simulink model "t_t_200_tge4"  (Simulink 6.2)
settings: Solver=ode45  StartTime=0.0  StopTime=10  RelTol=1e-3
undefined symbols (not defined in the file): BEE2_usr
libraries: xbsIndex_r3 x606, xps_library x57, casper_library x22
(part 2 of 4)

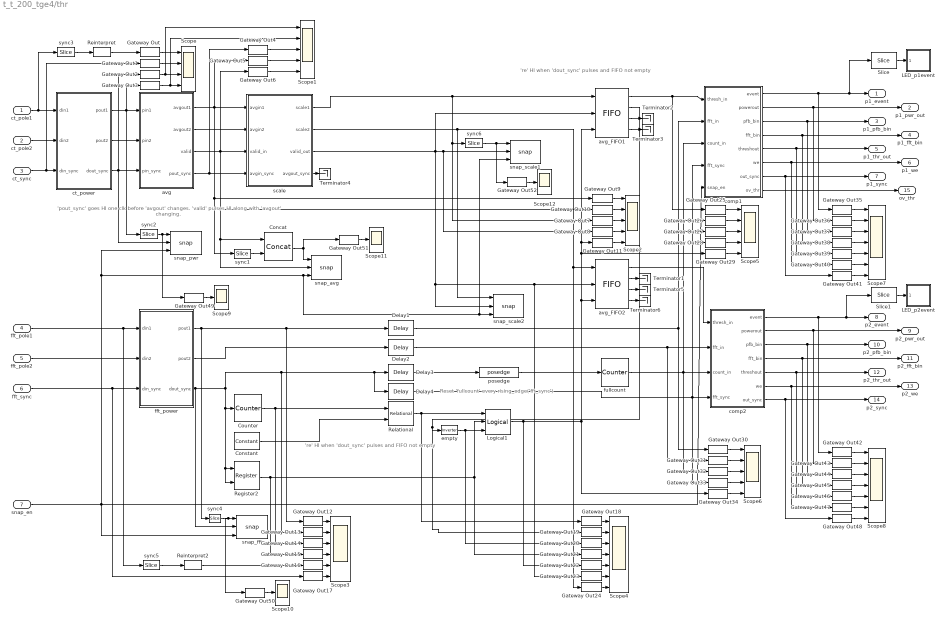
== system t_t_200_tge4/thr ==
  note: 'pout_sync' goes HI one clk
      | before 'avgout' changes.
      | 'valid' pulses HI along with
      | 'avgout' changing.
  note: 're' HI when 'dout_sync'
      | pulses and FIFO not empty
  note: 're' HI when 'dout_sync'
      | pulses and FIFO not empty
  note: Reset 'fullcount' every rising_edge('fft_sync')
  ct_pole1 : Inport  Port=1  LatchInput=off
  ct_pole2 : Inport  Port=2  LatchInput=off
  ct_sync : Inport  Port=3  LatchInput=off
  fft_pole1 : Inport  Port=4  LatchInput=off
  fft_pole2 : Inport  Port=5  LatchInput=off
  fft_sync : Inport  Port=6  LatchInput=off
  "snap_en " : Inport  Port=7  LatchInput=off
  Concat : xbsIndex_r3/Concat  num_inputs=2  explicit_period=off  period=1  dbl_ovrd=off
  Constant : xbsIndex_r3/Constant  const=0  equ=P=C  arith_type=Unsigned  n_bits=FFTSize  bin_pt=0  opselect=C  inp2=PCIN>>17  opr=+  inp1=P  carry=CIN  iostate=0  explicit_period=off  period=1  dbl_ovrd=off
  Counter : xbsIndex_r3/Counter  cnt_type=Free Running  n_bits=FFTSize  bin_pt=0  arith_type=Unsigned  start_count=0  cnt_to=Inf  cnt_by_val=1  operation=Up  explicit_period=off  period=1  load_pin=off  rst=on  en=off  dbl_ovrd=off  show_param=off  use_rpm=on  gen_core=off
      settings: xl_area=[0, 0, 0, 0, 0, 0, 0]
  Delay1 : xbsIndex_r3/Delay  latency=2  reg_retiming=off  explicit_period=off  period=1  en=off  accept_only_valid=off  init_zero=on  dbl_ovrd=off  show_param=off
      settings: xl_area=[0, 0, 0, 0, 0, 0, 0]
  Delay2 : xbsIndex_r3/Delay  latency=2  reg_retiming=off  explicit_period=off  period=1  en=off  accept_only_valid=off  init_zero=on  dbl_ovrd=off  show_param=off
      settings: xl_area=[0, 0, 0, 0, 0, 0, 0]
  Delay3 : xbsIndex_r3/Delay  latency=1  reg_retiming=off  explicit_period=off  period=1  en=off  accept_only_valid=off  init_zero=on  dbl_ovrd=off  show_param=off
      settings: xl_area=[0, 0, 0, 0, 0, 0, 0]
  Delay4 : xbsIndex_r3/Delay  latency=2  reg_retiming=off  explicit_period=off  period=1  en=off  accept_only_valid=off  init_zero=on  dbl_ovrd=off  show_param=off
      settings: xl_area=[0, 0, 0, 0, 0, 0, 0]
  Gateway Out{,1..52} (53 alike) : xbsIndex_r3/Gateway Out  output_type=Double  nbits=8  bin_pt=6  arith_type=Boolean  quantization=Truncate  overflow=Wrap  hdl_port=off  timing_constraint=None  locs_specified=off  LOCs={}  needs_fixed_name=off  show_param=off
      settings: xl_area=[0, 0, 0, 0, 0, 0, 0]
  LED_p1event : Subsystem  mask{pulse_length=200000}
      mask prompts: pulse_length "Pulse Length (samples)"
  LED_p2event : Subsystem  mask{pulse_length=200000}
      mask prompts: pulse_length "Pulse Length (samples)"
  Logical1 : xbsIndex_r3/Logical  logical_function=AND  inputs=3  precision=Full  arith_type=Unsigned  n_bits=8  bin_pt=2  align_bp=on  latency=0  explicit_period=off  period=1  en=off  dbl_ovrd=off  show_param=off
      settings: xl_area=[0, 0, 0, 0, 0, 0, 0]
  Register2 : xbsIndex_r3/Register  init=0  reg_only_valid=off  explicit_period=off  period=1  rst=off  en=on  out_en=off  dbl_ovrd=off  show_param=off
      settings: xl_area=[0, 0, 0, 0, 0, 0, 0]
  Reinterpret : xbsIndex_r3/Reinterpret  force_arith_type=on  arith_type="Signed  (2's comp)"  force_bin_pt=on  bin_pt=DataWidth-1  force_valid=on
  Reinterpret2 : xbsIndex_r3/Reinterpret  force_arith_type=on  arith_type="Signed  (2's comp)"  force_bin_pt=on  bin_pt=DataWidth-1  force_valid=on
  Relational : xbsIndex_r3/Relational  mode=a=b  latency=1  explicit_period=off  period=1  en=off  dbl_ovrd=off  show_param=off
      settings: xl_area=[0, 0, 0, 0, 0, 0, 0]
  Scope : Scope  NumInputPorts=4
      settings: YMin=-5~-5~-5~-5  YMax=5~5~5~5  SaveName=ScopeData9
  Scope{1..2,5..6} (4 alike) : Scope  NumInputPorts=5
      Scope1 settings: YMin=-5~-5~-5~-5~-5  YMax=5~5~5~5~5  SaveName=ScopeData10
      Scope2 settings: TimeRange=4300  YMin=-5~-5~-5~-5~-5  YMax=5~5~5~5~5  SaveName=ScopeData12
      Scope5 settings: YMin=-5~-5~-5~-5~-5  YMax=5~5~5~5~5  SaveName=ScopeData15
      Scope6 settings: YMin=-5~-5~-5~-5~-5  YMax=5~5~5~5~5  SaveName=ScopeData16
  Scope{9..12} (4 alike) : Scope
      Scope10 settings: YMin=8.97459e+008  YMax=9.91929e+008  SaveName=ScopeData23
      Scope11 settings: YMin=8.97459e+008  YMax=9.91929e+008  SaveName=ScopeData24
      Scope12 settings: YMin=8.97459e+008  YMax=9.91929e+008  SaveName=ScopeData25
      Scope9 settings: YMin=9.44694e+008  YMax=9.44694e+008  SaveName=ScopeData22
  Scope3 : Scope  NumInputPorts=6
      settings: YMin=-5~-5~-5~-5~-5~-5  YMax=5~5~5~5~5~5  SaveName=ScopeData13
  Scope4 : Scope  NumInputPorts=7
      settings: YMin=-5~-5~-5~-5~-5~-5~-5  YMax=5~5~5~5~5~5~5  SaveName=ScopeData14
  Scope7 : Scope  NumInputPorts=7
      settings: YMin=0~0~-1~0~0~0~0  YMax=1~1~1~1250~0.5~1~1  SaveName=ScopeData17
  Scope8 : Scope  NumInputPorts=7
      settings: YMin=-5~-5~-5~-5~-5~-5~-5  YMax=5~5~5~5~5~5~5  SaveName=ScopeData18
  Slice : xbsIndex_r3/Slice  mode=Lower Bit Location + Width  nbits=1  bit1=0  base1=MSB of Input  bit0=0  base0=LSB of Input  boolean_output=on  explicit_period=off  period=1  dbl_ovrd=off
  Slice1 : xbsIndex_r3/Slice  mode=Lower Bit Location + Width  nbits=1  bit1=0  base1=MSB of Input  bit0=0  base0=LSB of Input  boolean_output=on  explicit_period=off  period=1  dbl_ovrd=off
  Terminator{1..6} (6 alike) : Terminator
  avg : Subsystem  mask{FFTSize=FFTSize, DataWidth=DataWidth}
      mask prompts: FFTSize "FFT Size (2^?)"; DataWidth "Data Bitwidth"
  avg_FIFO1 : xbsIndex_r3/FIFO  depth=32  percent_nbits=1  store_only_valid=on  init_zero=on  explicit_period=off  period=1  rst=off  en=off  use_almost_empty=off  almost_empty_offset=6  use_almost_full=off  almost_full_offset=6  dbl_ovrd=off  show_param=off  mem_type=Block RAM  gen_core=off
      settings: xl_area=[0, 0, 0, 0, 0, 0, 0]
  avg_FIFO2 : xbsIndex_r3/FIFO  depth=32  percent_nbits=1  store_only_valid=on  init_zero=on  explicit_period=off  period=1  rst=off  en=off  use_almost_empty=off  almost_empty_offset=6  use_almost_full=off  almost_full_offset=6  dbl_ovrd=off  show_param=off  mem_type=Block RAM  gen_core=off
      settings: xl_area=[0, 0, 0, 0, 0, 0, 0]
  comp1 : Subsystem  mask{CPUWidth=CPUWidth, FFTSize=FFTSize, PFBSize=PFBSize}
      mask prompts: CPUWidth "CPU Bitwidth"; FFTSize "FFT Size (2^?)"; PFBSize "PFB Size  (2^?)"
  comp2 : Subsystem  mask{CPUWidth=CPUWidth, FFTSize=FFTSize, PFBSize=PFBSize}
      mask prompts: CPUWidth "CPU Bitwidth"; FFTSize "FFT Size (2^?)"; PFBSize "PFB Size  (2^?)"
  ct_power : Subsystem  mask{mult_lat=3, add_lat=2, DataWidth=DataWidth}
      mask prompts: mult_lat "Multiply Latency"; add_lat "Add Latency"; DataWidth "Data Width"
  empty : xbsIndex_r3/Inverter  latency=0  explicit_period=on  period=1  en=off  dbl_ovrd=off  show_param=off
      settings: xl_area=[0, 0, 0, 0, 0, 0, 0]
  fft_power : Subsystem  mask{mult_lat=3, add_lat=2, DataWidth=DataWidth}
      mask prompts: mult_lat "Multiply Latency"; add_lat "Add Latency"; DataWidth "Data Width"
  fullcount : xbsIndex_r3/Counter  cnt_type=Free Running  n_bits=FFTSize+PFBSize  bin_pt=0  arith_type=Unsigned  start_count=0  cnt_to=Inf  cnt_by_val=1  operation=Up  explicit_period=off  period=1  load_pin=off  rst=on  en=off  dbl_ovrd=off  show_param=off  use_rpm=on  gen_core=off
      settings: xl_area=[0, 0, 0, 0, 0, 0, 0]
  posedge : casper_library/Misc/posedge  Tag=Rising Edge Detector
  scale : Subsystem  mask{DataWidth=DataWidth, mult_lat=4, scale=1}
      mask prompts: DataWidth "Data Bitwidth"; mult_lat "Mulitply Latency"; scale "Test Scale"
  snap_avg : casper_library/Scopes/snap  nsamples=11
  snap_fft : casper_library/Scopes/snap  nsamples=11
  snap_pwr : casper_library/Scopes/snap  nsamples=11
  snap_scale1 : casper_library/Scopes/snap  nsamples=11
  snap_scale2 : casper_library/Scopes/snap  nsamples=11
  sync1 : xbsIndex_r3/Slice  mode=Lower Bit Location + Width  nbits=31  bit1=0  base1=MSB of Input  bit0=0  base0=LSB of Input  boolean_output=off  explicit_period=off  period=1  dbl_ovrd=off
  sync2 : xbsIndex_r3/Slice  mode=Lower Bit Location + Width  nbits=32  bit1=0  base1=MSB of Input  bit0=0  base0=LSB of Input  boolean_output=off  explicit_period=off  period=1  dbl_ovrd=off
  sync3 : xbsIndex_r3/Slice  mode=Lower Bit Location + Width  nbits=DataWidth  bit1=0  base1=MSB of Input  bit0=0  base0=LSB of Input  boolean_output=off  explicit_period=off  period=1  dbl_ovrd=off
  sync4 : xbsIndex_r3/Slice  mode=Lower Bit Location + Width  nbits=DataWidth  bit1=0  base1=MSB of Input  bit0=0  base0=LSB of Input  boolean_output=off  explicit_period=off  period=1  dbl_ovrd=off
  sync5 : xbsIndex_r3/Slice  mode=Lower Bit Location + Width  nbits=DataWidth  bit1=0  base1=MSB of Input  bit0=0  base0=LSB of Input  boolean_output=off  explicit_period=off  period=1  dbl_ovrd=off
  sync6 : xbsIndex_r3/Slice  mode=Lower Bit Location + Width  nbits=32  bit1=0  base1=MSB of Input  bit0=0  base0=LSB of Input  boolean_output=off  explicit_period=off  period=1  dbl_ovrd=off
  p1_event : Outport
  p1_pwr_out : Outport  Port=2
  p1_pfb_bin : Outport  Port=3
  p1_fft_bin : Outport  Port=4
  p1_thr_out : Outport  Port=5
  p1_we : Outport  Port=6
  p1_sync : Outport  Port=7
  p2_event : Outport  Port=8
  p2_pwr_out : Outport  Port=9
  p2_pfb_bin : Outport  Port=10
  p2_fft_bin : Outport  Port=11
  p2_thr_out : Outport  Port=12
  p2_we : Outport  Port=13
  p2_sync : Outport  Port=14
  ov_thr : Outport  Port=15
  wires:
  Slice1/1 -> LED_p2event/1(Sync_In)
  Gateway Out48/1 -> Scope8/7
  Gateway Out47/1 -> Scope8/6
  Gateway Out46/1 -> Scope8/5
  Gateway Out45/1 -> Scope8/4
  Gateway Out44/1 -> Scope8/3
  Gateway Out43/1 -> Scope8/2
  Gateway Out42/1 -> Scope8/1
  Gateway Out41/1 -> Scope7/7
  Gateway Out40/1 -> Scope7/6
  Gateway Out39/1 -> Scope7/5
  Gateway Out38/1 -> Scope7/4
  Gateway Out37/1 -> Scope7/3
  Gateway Out36/1 -> Scope7/2
  Gateway Out35/1 -> Scope7/1
  Gateway Out34/1 -> Scope6/5
  Gateway Out33/1 -> Scope6/4
  Gateway Out32/1 -> Scope6/3
  Gateway Out31/1 -> Scope6/2
  Gateway Out30/1 -> Scope6/1
  Gateway Out29/1 -> Scope5/5
  Gateway Out28/1 -> Scope5/4
  Gateway Out27/1 -> Scope5/3
  Gateway Out26/1 -> Scope5/2
  Gateway Out25/1 -> Scope5/1
  Gateway Out24/1 -> Scope4/7
  Gateway Out23/1 -> Scope4/6
  Gateway Out22/1 -> Scope4/5
  Gateway Out21/1 -> Scope4/4
  Gateway Out20/1 -> Scope4/3
  Gateway Out19/1 -> Scope4/2
  Gateway Out18/1 -> Scope4/1
  Gateway Out17/1 -> Scope3/6
  Gateway Out16/1 -> Scope3/5
  Gateway Out15/1 -> Scope3/4
  Gateway Out14/1 -> Scope3/3
  Gateway Out13/1 -> Scope3/2
  Gateway Out12/1 -> Scope3/1
  Gateway Out11/1 -> Scope2/5
  Gateway Out8/1 -> Scope2/4
  Gateway Out7/1 -> Scope2/3
  Gateway Out10/1 -> Scope2/2
  Gateway Out9/1 -> Scope2/1
  Gateway Out4/1 -> Scope1/3
  Gateway Out5/1 -> Scope1/4
  Gateway Out6/1 -> Scope1/5
  Gateway Out3/1 -> Scope/4, Scope1/2
  Gateway Out2/1 -> Scope/3, Scope1/1
  Gateway Out1/1 -> Scope/2
  Gateway Out/1 -> Scope/1
  Reinterpret/1 -> Gateway Out/1
  sync3/1 -> Reinterpret/1
  ct_sync/1 -> Gateway Out1/1, ct_power/3(din_sync)
  scale/1(scale1) -> Gateway Out7/1, sync6/1, avg_FIFO1/1
  sync2/1 -> snap_pwr/1, Gateway Out49/1
  comp1/6(we) -> p1_we/1, Gateway Out40/1
  comp1/1(event) -> Gateway Out35/1, Slice/1, p1_event/1
  sync1/1 -> Concat/2
  Concat/1 -> snap_avg/1, Gateway Out51/1
  "snap_en "/1 -> snap_pwr/3, snap_avg/3, snap_scale2/3, snap_scale1/3, comp1/5("snap_en "), snap_fft/3
  scale/4(avgout_sync) -> Terminator4/1
  empty/1 -> Gateway Out20/1, Logical1/3
  Logical1/1 -> Gateway Out22/1, Gateway Out34/1, Gateway Out29/1, Gateway Out11/1, avg_FIFO1/3, avg_FIFO2/3
  avg_FIFO1/2 -> Gateway Out19/1, empty/1
  avg/4(pout_sync) -> Gateway Out4/1, scale/4(avgin_sync)
  Delay2/1 -> comp2/2(fft_in), Gateway Out31/1
  Slice/1 -> LED_p1event/1(Sync_In)
  avg/3(valid) -> Gateway Out10/1, Concat/1, snap_avg/2, Gateway Out6/1, scale/3(valid_in)
  Relational/1 -> Gateway Out18/1, Logical1/1
  Register2/1 -> Gateway Out21/1, Logical1/2, Gateway Out15/1
  fft_sync/1 -> Gateway Out17/1, fft_power/3(din_sync)
  fft_pole2/1 -> fft_power/2(din2)
  fft_pole1/1 -> fft_power/1(din1), sync5/1
  ct_pole2/1 -> ct_power/2(din2)
  ct_pole1/1 -> sync3/1, ct_power/1(din1)
  comp2/7(out_sync) -> Gateway Out48/1, p2_sync/1
  comp2/6(we) -> Gateway Out47/1, p2_we/1
  comp2/5(threshout) -> Gateway Out46/1, p2_thr_out/1
  comp2/4(fft_bin) -> Gateway Out45/1, p2_fft_bin/1
  comp2/3(pfb_bin) -> Gateway Out44/1, p2_pfb_bin/1
  comp2/2(powerout) -> Gateway Out43/1, p2_pwr_out/1
  comp2/1(event) -> Slice1/1, p2_event/1, Gateway Out42/1
  comp1/7(out_sync) -> Gateway Out41/1, p1_sync/1
  comp1/5(threshout) -> Gateway Out39/1, p1_thr_out/1
  comp1/4(fft_bin) -> Gateway Out38/1, p1_fft_bin/1
  comp1/3(pfb_bin) -> Gateway Out37/1, p1_pfb_bin/1
  comp1/2(powerout) -> Gateway Out36/1, p1_pwr_out/1
  Delay1/1 -> Gateway Out30/1, Gateway Out26/1, comp1/2(fft_in)
  fullcount/1 -> comp2/3(count_in), Gateway Out32/1, Gateway Out27/1, comp1/3(count_in)
  fft_power/2(pout2) -> Delay2/1
  avg_FIFO2/4 -> Terminator6/1
  avg_FIFO2/3 -> Terminator5/1
  avg_FIFO1/4 -> Terminator3/1
  avg_FIFO1/3 -> Terminator2/1
  avg_FIFO2/1 -> comp2/1(thresh_in)
  fft_power/1(pout1) -> Gateway Out12/1, Delay1/1, sync4/1
  avg_FIFO1/1 -> Gateway Out25/1, comp1/1(thresh_in)
  fft_power/3(dout_sync) -> Gateway Out13/1, Delay3/1, Delay4/1, Counter/1, Register2/1, Register2/2, snap_fft/2
  Constant/1 -> Relational/2
  Counter/1 -> Gateway Out14/1, Relational/1
  scale/3(valid_out) -> Gateway Out8/1, snap_scale1/2, avg_FIFO1/2, Gateway Out23/1, avg_FIFO2/2, snap_scale2/2
  scale/2(scale2) -> Gateway Out24/1, avg_FIFO2/1, snap_scale2/1
  avg/2(avgout2) -> scale/2(avgin2)
  avg/1(avgout1) -> Gateway Out9/1, sync1/1, Gateway Out5/1, scale/1(avgin1)
  ct_power/3(dout_sync) -> Gateway Out2/1, avg/3(pin_sync), snap_pwr/2
  ct_power/2(pout2) -> avg/2(pin2)
  ct_power/1(pout1) -> Gateway Out3/1, sync2/1, avg/1(pin1)
  sync5/1 -> Reinterpret2/1
  Reinterpret2/1 -> Gateway Out16/1
  Delay3/1 -> posedge/1
  posedge/1 -> fullcount/1
  Delay4/1 -> comp2/4(fft_sync), Gateway Out33/1, comp1/4(fft_sync), Gateway Out28/1
  Gateway Out49/1 -> Scope9/1
  sync4/1 -> snap_fft/1, Gateway Out50/1
  Gateway Out50/1 -> Scope10/1
  Gateway Out51/1 -> Scope11/1
  sync6/1 -> snap_scale1/1, Gateway Out52/1
  Gateway Out52/1 -> Scope12/1
  comp1/8(ov_thr) -> ov_thr/1
  avg_FIFO2/2 -> Terminator1/1

== system t_t_200_tge4/ct_in_mux/concat ==
  In1 : Inport  Orientation=down  Port=1  LatchInput=off
  Concat : xbsIndex_r3/Concat  num_inputs=4  explicit_period=on  period=1  dbl_ovrd=off
  Constant : xbsIndex_r3/Constant  const=0  equ=P=C  arith_type=Unsigned  n_bits=14  bin_pt=0  opselect=C  inp2=PCIN>>17  opr=+  inp1=P  carry=CIN  iostate=0  explicit_period=on  period=1  dbl_ovrd=off
  Slice3 : xbsIndex_r3/Slice  mode=Upper Bit Location + Width  nbits=18  bit1=0  base1=MSB of Input  bit0=0  base0=LSB of Input  boolean_output=off  explicit_period=off  period=1  dbl_ovrd=off
  Slice4 : xbsIndex_r3/Slice  mode=Lower Bit Location + Width  nbits=18  bit1=0  base1=MSB of Input  bit0=0  base0=LSB of Input  boolean_output=off  explicit_period=off  period=1  dbl_ovrd=off
  Out1 : Outport
  wires:
  Slice3/1 -> Concat/2
  Constant/1 -> Concat/1, Concat/3
  Slice4/1 -> Concat/4
  In1/1 -> Slice3/1, Slice4/1
  Concat/1 -> Out1/1

== system t_t_200_tge4/ct_in_mux/trig_delay ==
  data_in : Inport  Port=1  LatchInput=off
  trig_in : Inport  Port=2  LatchInput=off
  delay : Inport  Port=3  LatchInput=off
  Constant : xbsIndex_r3/Constant  const=1  equ=P=C  arith_type=Boolean  n_bits=32  bin_pt=0  opselect=C  inp2=PCIN>>17  opr=+  inp1=P  carry=CIN  iostate=0  explicit_period=on  period=1  dbl_ovrd=off
  Counter : xbsIndex_r3/Counter  cnt_type=Free Running  n_bits=32  bin_pt=0  arith_type=Unsigned  start_count=0  cnt_to=Inf  cnt_by_val=1  operation=Up  explicit_period=on  period=1  load_pin=off  rst=on  en=on  dbl_ovrd=off  show_param=off  use_rpm=on  gen_core=off
      settings: xl_area=[0, 0, 0, 0, 0, 0, 0]
  Delay : xbsIndex_r3/Delay  latency=2  reg_retiming=off  explicit_period=on  period=1  en=off  accept_only_valid=off  init_zero=on  dbl_ovrd=off  show_param=off
      settings: xl_area=[0, 0, 0, 0, 0, 0, 0]
  Gateway Out : xbsIndex_r3/Gateway Out  output_type=Double  nbits=8  bin_pt=6  arith_type=Boolean  quantization=Truncate  overflow=Wrap  hdl_port=on  timing_constraint=None  locs_specified=off  LOCs={}  needs_fixed_name=off  show_param=off
      settings: xl_area=[0, 0, 0, 0, 0, 0, 0]
  Gateway Out1 : xbsIndex_r3/Gateway Out  output_type=Double  nbits=8  bin_pt=6  arith_type=Boolean  quantization=Truncate  overflow=Wrap  hdl_port=on  timing_constraint=None  locs_specified=off  LOCs={}  needs_fixed_name=off  show_param=off
      settings: xl_area=[0, 0, 0, 0, 0, 0, 0]
  Register : xbsIndex_r3/Register  init=0  reg_only_valid=off  explicit_period=on  period=1  rst=on  en=on  out_en=off  dbl_ovrd=off  show_param=off
      settings: xl_area=[0, 0, 0, 0, 0, 0, 0]
  Relational : xbsIndex_r3/Relational  mode=a=b  latency=1  explicit_period=on  period=1  en=on  dbl_ovrd=off  show_param=off
      settings: xl_area=[0, 0, 0, 0, 0, 0, 0]
  Scope : Scope  NumInputPorts=2
      settings: YMin=-5~-5  YMax=5~5
  posedge : casper_library/Misc/posedge  Tag=Rising Edge Detector
  data_out : Outport
  trig_out : Outport  Port=2
  wires:
  delay/1 -> Relational/1
  trig_in/1 -> Register/3, Gateway Out1/1
  Constant/1 -> Register/1
  Relational/1 -> Register/2, Counter/1, Gateway Out/1, posedge/1
  Register/1 -> Counter/2, Relational/3
  Counter/1 -> Relational/2
  Gateway Out/1 -> Scope/1
  Gateway Out1/1 -> Scope/2
  data_in/1 -> Delay/1
  Delay/1 -> data_out/1
  posedge/1 -> trig_out/1

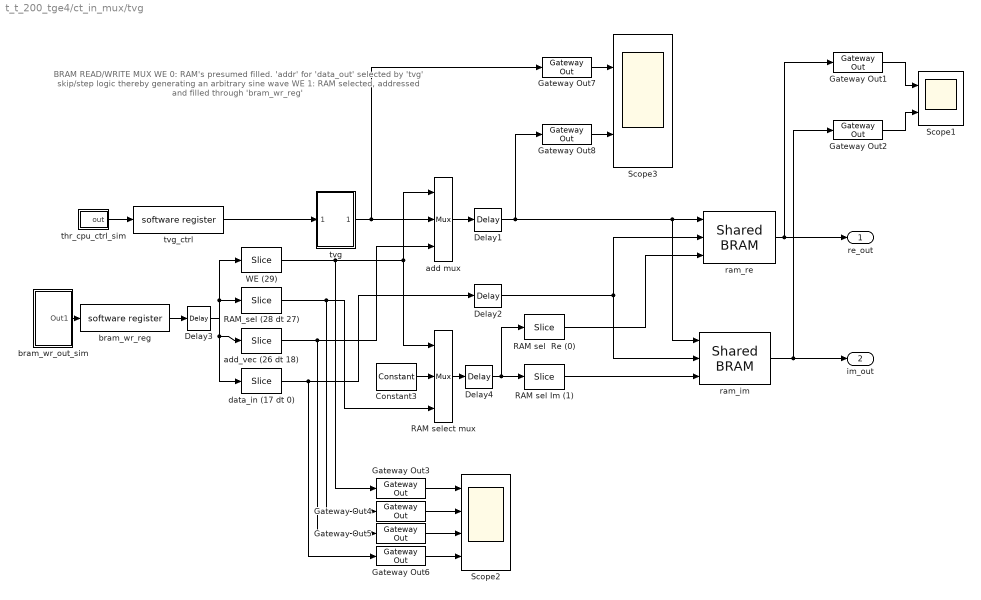
== system t_t_200_tge4/ct_in_mux/tvg ==
  note: BRAM READ/WRITE MUX
      | WE 0: RAM's presumed filled.
      | 'addr' for 'data_out' selected
      | by 'tvg' skip/step logic thereby
      | generating an arbitrary sine wave
      | WE 1: RAM selected, addressed
      | and filled through
      | 'bram_wr_reg'
  Constant3 : xbsIndex_r3/Constant  const=0  equ=P=C  arith_type=Unsigned  n_bits=4  bin_pt=0  opselect=C  inp2=PCIN>>17  opr=+  inp1=P  carry=CIN  iostate=0  explicit_period=on  period=1  dbl_ovrd=off
  Delay{1..4} (4 alike) : xbsIndex_r3/Delay  latency=1  reg_retiming=on  explicit_period=on  period=1  en=off  accept_only_valid=off  init_zero=on  dbl_ovrd=off  show_param=off
      settings: xl_area=[0, 0, 0, 0, 0, 0, 0]
  Gateway Out{1..8} (8 alike) : xbsIndex_r3/Gateway Out  output_type=Double  nbits=8  bin_pt=6  arith_type=Boolean  quantization=Truncate  overflow=Wrap  hdl_port=on  timing_constraint=None  locs_specified=off  LOCs={}  needs_fixed_name=off  show_param=off
      settings: xl_area=[0, 0, 0, 0, 0, 0, 0]
  RAM sel  Re (0) : xbsIndex_r3/Slice  mode=Lower Bit Location + Width  nbits=1  bit1=0  base1=MSB of Input  bit0=0  base0=LSB of Input  boolean_output=on  explicit_period=on  period=1  dbl_ovrd=off
  RAM sel Im (1) : xbsIndex_r3/Slice  mode=Lower Bit Location + Width  nbits=1  bit1=0  base1=MSB of Input  bit0=1  base0=LSB of Input  boolean_output=on  explicit_period=on  period=1  dbl_ovrd=off
  RAM select mux : xbsIndex_r3/Mux  inputs=2  precision=Full  arith_type="Signed  (2's comp)"  n_bits=8  bin_pt=2  quantization=Truncate  overflow=Wrap  latency=0  explicit_period=on  period=1  en=off  dbl_ovrd=off  show_param=off  mux_type=off  use_rpm=off  gen_core=off
      settings: xl_area=[0, 0, 0, 0, 0, 0, 0]
  RAM_sel (28 dt 27) : xbsIndex_r3/Slice  mode=Lower Bit Location + Width  nbits=2  bit1=10  base1=MSB of Input  bit0=27  base0=LSB of Input  boolean_output=off  explicit_period=on  period=1  dbl_ovrd=off
  Scope1 : Scope  NumInputPorts=2
      settings: YMin=-5~-5  YMax=5~5  SaveName=ScopeData2
  Scope2 : Scope  NumInputPorts=4
      settings: YMin=-5~-5~-5~-5  YMax=5~5~5~5
  Scope3 : Scope  NumInputPorts=2
      settings: YMin=-5~-5  YMax=5~5  SaveName=ScopeData3
  WE (29) : xbsIndex_r3/Slice  mode=Lower Bit Location + Width  nbits=1  bit1=10  base1=MSB of Input  bit0=29  base0=LSB of Input  boolean_output=off  explicit_period=on  period=1  dbl_ovrd=off
  add mux : xbsIndex_r3/Mux  inputs=2  precision=Full  arith_type="Signed  (2's comp)"  n_bits=8  bin_pt=2  quantization=Truncate  overflow=Wrap  latency=0  explicit_period=on  period=1  en=off  dbl_ovrd=off  show_param=off  mux_type=off  use_rpm=off  gen_core=off
      settings: xl_area=[0, 0, 0, 0, 0, 0, 0]
  add_vec (26 dt 18) : xbsIndex_r3/Slice  mode=Lower Bit Location + Width  nbits=9  bit1=0  base1=MSB of Input  bit0=18  base0=LSB of Input  boolean_output=off  explicit_period=on  period=1  dbl_ovrd=off
  bram_wr_out_sim : Subsystem  mask{we_enable=0, ram_sel=3, add_vec=512, data_in=32}
      mask prompts: we_enable "Write enable"; ram_sel "RAM selector (1 = Re; 2 = Im; 3 = both)"; add_vec "RAM address"; data_in "Data in"
  bram_wr_reg : xps_library/software register  Tag=xps:sw_reg  io_dir=From Processor  arith_type=Unsigned  bitwidth=32  bin_pt=0  sample_period=1  gw_name=t_t_200_tge4_ct_in_mux_tvg_bram_wr_reg_user_data_out
  data_in (17 dt 0) : xbsIndex_r3/Slice  mode=Lower Bit Location + Width  nbits=18  bit1=0  base1=MSB of Input  bit0=0  base0=LSB of Input  boolean_output=off  explicit_period=on  period=1  dbl_ovrd=off
  ram_im : xps_library/Shared BRAM  Tag=xps:bram  arith_type="Signed  (2's comp)"  addr_width=11  data_width=32  data_bin_pt=0  init_vals=[1:2^11]  sample_rate=1
  ram_re : xps_library/Shared BRAM  Tag=xps:bram  arith_type="Signed  (2's comp)"  addr_width=11  data_width=32  data_bin_pt=0  init_vals=[1:2^11]  sample_rate=1
  thr_cpu_ctrl_sim : Subsystem  mask{tvg_skip=1, tvg_stall=2, tvg_length=5}
      mask prompts: tvg_skip "Skip"; tvg_stall "Stall"; tvg_length "Length"
      mask help:
      | Mux Data for CT and FFT Syncs:
      |
      | 0 -> Interchip Connection
      | 1 -> User Generated External Sync
      | 2 -> Periodic Sync Generator
      | 3 -> Periodic Sync Generator (Same as 2)
      |
      | Mux Data for CT and FFT Inputs:
      |
      | 0 -> Interchip Connection
      | 1 -> Test Vector Generator (TVG)
      | 2 -> All Zeroes (0's)
      | 3 -> All Ones (1's)
  tvg : Subsystem  mask(Test Vector Generator(TVG)){tvg_skip=1, tvg_stall=1, tvg_length=512}
      mask prompts: tvg_skip "Skip"; tvg_stall "Stall"; tvg_length "Length"
  tvg_ctrl : xps_library/software register  Tag=xps:sw_reg  io_dir=From Processor  arith_type=Unsigned  bitwidth=32  bin_pt=0  sample_period=1  gw_name=t_t_200_tge4_ct_in_mux_tvg_tvg_ctrl_user_data_out
  re_out : Outport
  im_out : Outport  Port=2
  wires:
  Delay3/1 -> RAM_sel (28 dt 27)/1, WE (29)/1, add_vec (26 dt 18)/1, data_in (17 dt 0)/1
  bram_wr_reg/1 -> Delay3/1
  tvg_ctrl/1 -> tvg/1(In1)
  tvg/1(Out1) -> add mux/2, Gateway Out7/1
  Constant3/1 -> RAM select mux/2
  RAM select mux/1 -> Delay4/1
  RAM sel  Re (0)/1 -> ram_re/3
  Gateway Out1/1 -> Scope1/1
  Gateway Out2/1 -> Scope1/2
  thr_cpu_ctrl_sim/1(out) -> tvg_ctrl/1
  add_vec (26 dt 18)/1 -> Gateway Out5/1, add mux/3
  RAM_sel (28 dt 27)/1 -> Gateway Out4/1, RAM select mux/3
  add mux/1 -> Delay1/1
  data_in (17 dt 0)/1 -> Gateway Out6/1, Delay2/1
  RAM sel Im (1)/1 -> ram_im/3
  ram_re/1 -> Gateway Out1/1, re_out/1
  ram_im/1 -> Gateway Out2/1, im_out/1
  bram_wr_out_sim/1(Out1) -> bram_wr_reg/1
  Gateway Out3/1 -> Scope2/1
  Gateway Out4/1 -> Scope2/2
  Gateway Out5/1 -> Scope2/3
  Gateway Out6/1 -> Scope2/4
  WE (29)/1 -> Gateway Out3/1, add mux/1, RAM select mux/1
  Gateway Out7/1 -> Scope3/1
  Gateway Out8/1 -> Scope3/2
  Delay1/1 -> ram_im/1, ram_re/1, Gateway Out8/1
  Delay2/1 -> ram_re/2, ram_im/2
  Delay4/1 -> RAM sel  Re (0)/1, RAM sel Im (1)/1

== system t_t_200_tge4/fft_in_mux/concat ==
  In1 : Inport  Port=1  LatchInput=off
  Concat : xbsIndex_r3/Concat  num_inputs=4  explicit_period=on  period=1  dbl_ovrd=off
  Constant : xbsIndex_r3/Constant  const=0  equ=P=C  arith_type=Unsigned  n_bits=14  bin_pt=0  opselect=C  inp2=PCIN>>17  opr=+  inp1=P  carry=CIN  iostate=0  explicit_period=on  period=1  dbl_ovrd=off
  Slice3 : xbsIndex_r3/Slice  mode=Upper Bit Location + Width  nbits=18  bit1=0  base1=MSB of Input  bit0=0  base0=LSB of Input  boolean_output=off  explicit_period=off  period=1  dbl_ovrd=off
  Slice4 : xbsIndex_r3/Slice  mode=Lower Bit Location + Width  nbits=18  bit1=0  base1=MSB of Input  bit0=0  base0=LSB of Input  boolean_output=off  explicit_period=off  period=1  dbl_ovrd=off
  Out1 : Outport
  wires:
  Slice4/1 -> Concat/4
  Slice3/1 -> Concat/2
  Constant/1 -> Concat/1, Concat/3
  In1/1 -> Slice4/1, Slice3/1
  Concat/1 -> Out1/1

== system t_t_200_tge4/fft_in_mux/trig_delay ==
  data_in : Inport  Port=1  LatchInput=off
  trig_in : Inport  Port=2  LatchInput=off
  delay : Inport  Port=3  LatchInput=off
  Constant : xbsIndex_r3/Constant  const=1  equ=P=C  arith_type=Boolean  n_bits=32  bin_pt=0  opselect=C  inp2=PCIN>>17  opr=+  inp1=P  carry=CIN  iostate=0  explicit_period=on  period=1  dbl_ovrd=off
  Counter : xbsIndex_r3/Counter  cnt_type=Free Running  n_bits=32  bin_pt=0  arith_type=Unsigned  start_count=0  cnt_to=Inf  cnt_by_val=1  operation=Up  explicit_period=on  period=1  load_pin=off  rst=on  en=on  dbl_ovrd=off  show_param=off  use_rpm=on  gen_core=off
      settings: xl_area=[0, 0, 0, 0, 0, 0, 0]
  Delay : xbsIndex_r3/Delay  latency=2  reg_retiming=off  explicit_period=on  period=1  en=off  accept_only_valid=off  init_zero=on  dbl_ovrd=off  show_param=off
      settings: xl_area=[0, 0, 0, 0, 0, 0, 0]
  Gateway Out : xbsIndex_r3/Gateway Out  output_type=Double  nbits=8  bin_pt=6  arith_type=Boolean  quantization=Truncate  overflow=Wrap  hdl_port=on  timing_constraint=None  locs_specified=off  LOCs={}  needs_fixed_name=off  show_param=off
      settings: xl_area=[0, 0, 0, 0, 0, 0, 0]
  Gateway Out1 : xbsIndex_r3/Gateway Out  output_type=Double  nbits=8  bin_pt=6  arith_type=Boolean  quantization=Truncate  overflow=Wrap  hdl_port=on  timing_constraint=None  locs_specified=off  LOCs={}  needs_fixed_name=off  show_param=off
      settings: xl_area=[0, 0, 0, 0, 0, 0, 0]
  Register : xbsIndex_r3/Register  init=0  reg_only_valid=off  explicit_period=on  period=1  rst=on  en=on  out_en=off  dbl_ovrd=off  show_param=off
      settings: xl_area=[0, 0, 0, 0, 0, 0, 0]
  Relational : xbsIndex_r3/Relational  mode=a=b  latency=1  explicit_period=on  period=1  en=on  dbl_ovrd=off  show_param=off
      settings: xl_area=[0, 0, 0, 0, 0, 0, 0]
  Scope : Scope  NumInputPorts=2
      settings: YMin=-5~-5  YMax=5~5
  posedge : casper_library/Misc/posedge  Tag=Rising Edge Detector
  data_out : Outport
  trig_out : Outport  Port=2
  wires:
  delay/1 -> Relational/1
  trig_in/1 -> Register/3, Gateway Out1/1
  Constant/1 -> Register/1
  Relational/1 -> Register/2, Counter/1, Gateway Out/1, posedge/1
  Register/1 -> Counter/2, Relational/3
  Counter/1 -> Relational/2
  Gateway Out/1 -> Scope/1
  Gateway Out1/1 -> Scope/2
  data_in/1 -> Delay/1
  Delay/1 -> data_out/1
  posedge/1 -> trig_out/1

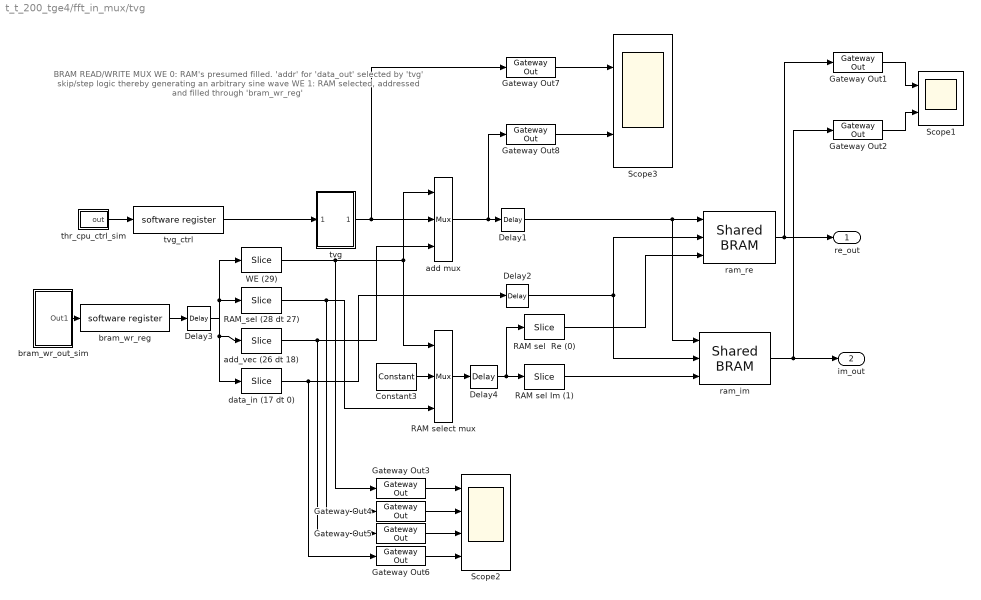
== system t_t_200_tge4/fft_in_mux/tvg ==
  note: BRAM READ/WRITE MUX
      | WE 0: RAM's presumed filled.
      | 'addr' for 'data_out' selected
      | by 'tvg' skip/step logic thereby
      | generating an arbitrary sine wave
      | WE 1: RAM selected, addressed
      | and filled through
      | 'bram_wr_reg'
  Constant3 : xbsIndex_r3/Constant  const=0  equ=P=C  arith_type=Unsigned  n_bits=4  bin_pt=0  opselect=C  inp2=PCIN>>17  opr=+  inp1=P  carry=CIN  iostate=0  explicit_period=on  period=1  dbl_ovrd=off
  Delay{1..4} (4 alike) : xbsIndex_r3/Delay  latency=1  reg_retiming=on  explicit_period=on  period=1  en=off  accept_only_valid=off  init_zero=on  dbl_ovrd=off  show_param=off
      settings: xl_area=[0, 0, 0, 0, 0, 0, 0]
  Gateway Out{1..8} (8 alike) : xbsIndex_r3/Gateway Out  output_type=Double  nbits=8  bin_pt=6  arith_type=Boolean  quantization=Truncate  overflow=Wrap  hdl_port=on  timing_constraint=None  locs_specified=off  LOCs={}  needs_fixed_name=off  show_param=off
      settings: xl_area=[0, 0, 0, 0, 0, 0, 0]
  RAM sel  Re (0) : xbsIndex_r3/Slice  mode=Lower Bit Location + Width  nbits=1  bit1=0  base1=MSB of Input  bit0=0  base0=LSB of Input  boolean_output=on  explicit_period=on  period=1  dbl_ovrd=off
  RAM sel Im (1) : xbsIndex_r3/Slice  mode=Lower Bit Location + Width  nbits=1  bit1=0  base1=MSB of Input  bit0=1  base0=LSB of Input  boolean_output=on  explicit_period=on  period=1  dbl_ovrd=off
  RAM select mux : xbsIndex_r3/Mux  inputs=2  precision=Full  arith_type="Signed  (2's comp)"  n_bits=8  bin_pt=2  quantization=Truncate  overflow=Wrap  latency=0  explicit_period=on  period=1  en=off  dbl_ovrd=off  show_param=off  mux_type=off  use_rpm=off  gen_core=off
      settings: xl_area=[0, 0, 0, 0, 0, 0, 0]
  RAM_sel (28 dt 27) : xbsIndex_r3/Slice  mode=Lower Bit Location + Width  nbits=2  bit1=10  base1=MSB of Input  bit0=27  base0=LSB of Input  boolean_output=off  explicit_period=on  period=1  dbl_ovrd=off
  Scope1 : Scope  NumInputPorts=2
      settings: YMin=-5~-5  YMax=5~5  SaveName=ScopeData2
  Scope2 : Scope  NumInputPorts=4
      settings: YMin=-5~-5~-5~-5  YMax=5~5~5~5
  Scope3 : Scope  NumInputPorts=2
      settings: YMin=-5~-5  YMax=5~5  SaveName=ScopeData3
  WE (29) : xbsIndex_r3/Slice  mode=Lower Bit Location + Width  nbits=1  bit1=10  base1=MSB of Input  bit0=29  base0=LSB of Input  boolean_output=off  explicit_period=on  period=1  dbl_ovrd=off
  add mux : xbsIndex_r3/Mux  inputs=2  precision=Full  arith_type="Signed  (2's comp)"  n_bits=8  bin_pt=2  quantization=Truncate  overflow=Wrap  latency=0  explicit_period=on  period=1  en=off  dbl_ovrd=off  show_param=off  mux_type=off  use_rpm=off  gen_core=off
      settings: xl_area=[0, 0, 0, 0, 0, 0, 0]
  add_vec (26 dt 18) : xbsIndex_r3/Slice  mode=Lower Bit Location + Width  nbits=9  bit1=0  base1=MSB of Input  bit0=18  base0=LSB of Input  boolean_output=off  explicit_period=on  period=1  dbl_ovrd=off
  bram_wr_out_sim : Subsystem  mask{we_enable=0, ram_sel=3, add_vec=512, data_in=32}
      mask prompts: we_enable "Write enable"; ram_sel "RAM selector (1 = Re; 2 = Im; 3 = both)"; add_vec "RAM address"; data_in "Data in"
  bram_wr_reg : xps_library/software register  Tag=xps:sw_reg  io_dir=From Processor  arith_type=Unsigned  bitwidth=32  bin_pt=0  sample_period=1  gw_name=t_t_200_tge4_fft_in_mux_tvg_bram_wr_reg_user_data_out
  data_in (17 dt 0) : xbsIndex_r3/Slice  mode=Lower Bit Location + Width  nbits=18  bit1=0  base1=MSB of Input  bit0=0  base0=LSB of Input  boolean_output=off  explicit_period=on  period=1  dbl_ovrd=off
  ram_im : xps_library/Shared BRAM  Tag=xps:bram  arith_type="Signed  (2's comp)"  addr_width=11  data_width=32  data_bin_pt=0  init_vals=[1:2^11]  sample_rate=1
  ram_re : xps_library/Shared BRAM  Tag=xps:bram  arith_type="Signed  (2's comp)"  addr_width=11  data_width=32  data_bin_pt=0  init_vals=[1:2^11]  sample_rate=1
  thr_cpu_ctrl_sim : Subsystem  mask{tvg_skip=1, tvg_stall=2, tvg_length=5}
      mask prompts: tvg_skip "Skip"; tvg_stall "Stall"; tvg_length "Length"
      mask help:
      | Mux Data for CT and FFT Syncs:
      |
      | 0 -> Interchip Connection
      | 1 -> User Generated External Sync
      | 2 -> Periodic Sync Generator
      | 3 -> Periodic Sync Generator (Same as 2)
      |
      | Mux Data for CT and FFT Inputs:
      |
      | 0 -> Interchip Connection
      | 1 -> Test Vector Generator (TVG)
      | 2 -> All Zeroes (0's)
      | 3 -> All Ones (1's)
  tvg : Subsystem  mask(Test Vector Generator(TVG)){tvg_skip=1, tvg_stall=1, tvg_length=512}
      mask prompts: tvg_skip "Skip"; tvg_stall "Stall"; tvg_length "Length"
  tvg_ctrl : xps_library/software register  Tag=xps:sw_reg  io_dir=From Processor  arith_type=Unsigned  bitwidth=32  bin_pt=0  sample_period=1  gw_name=t_t_200_tge4_fft_in_mux_tvg_tvg_ctrl_user_data_out
  re_out : Outport
  im_out : Outport  Port=2
  wires:
  Delay3/1 -> RAM_sel (28 dt 27)/1, WE (29)/1, add_vec (26 dt 18)/1, data_in (17 dt 0)/1
  bram_wr_reg/1 -> Delay3/1
  tvg_ctrl/1 -> tvg/1(In1)
  tvg/1(Out1) -> add mux/2, Gateway Out7/1
  Constant3/1 -> RAM select mux/2
  RAM select mux/1 -> Delay4/1
  RAM sel  Re (0)/1 -> ram_re/3
  Gateway Out1/1 -> Scope1/1
  Gateway Out2/1 -> Scope1/2
  thr_cpu_ctrl_sim/1(out) -> tvg_ctrl/1
  add_vec (26 dt 18)/1 -> Gateway Out5/1, add mux/3
  RAM_sel (28 dt 27)/1 -> Gateway Out4/1, RAM select mux/3
  add mux/1 -> Gateway Out8/1, Delay1/1
  data_in (17 dt 0)/1 -> Gateway Out6/1, Delay2/1
  RAM sel Im (1)/1 -> ram_im/3
  ram_re/1 -> Gateway Out1/1, re_out/1
  ram_im/1 -> Gateway Out2/1, im_out/1
  bram_wr_out_sim/1(Out1) -> bram_wr_reg/1
  Gateway Out3/1 -> Scope2/1
  Gateway Out4/1 -> Scope2/2
  Gateway Out5/1 -> Scope2/3
  Gateway Out6/1 -> Scope2/4
  WE (29)/1 -> Gateway Out3/1, add mux/1, RAM select mux/1
  Gateway Out7/1 -> Scope3/1
  Gateway Out8/1 -> Scope3/2
  Delay1/1 -> ram_im/1, ram_re/1
  Delay2/1 -> ram_re/2, ram_im/2
  Delay4/1 -> RAM sel  Re (0)/1, RAM sel Im (1)/1

== system t_t_200_tge4/rec/LED_fifo2we ==
  Sync_In : Inport  Port=1  LatchInput=off
  Scope : Scope
  gpio : xps_library/gpio  Tag=xps:gpio  io_group=BEE2_usr:led  io_dir=out  arith_type=Boolean  bitwidth=1  bin_pt=0  bit_index=5  sample_period=1  use_single_ended=off  use_ddr=off  reg_iob=on  reg_clk_phase=0  termination=None
  wires:
  gpio/1 -> Scope/1
  Sync_In/1 -> gpio/1

== system t_t_200_tge4/rec/reg_once ==
  d : Inport  Port=1  LatchInput=off
  en : Inport  Port=2  LatchInput=off
  Convert : xbsIndex_r3/Convert  arith_type=Boolean  n_bits=8  bin_pt=6  quantization=Truncate  overflow=Wrap  latency=0  explicit_period=off  period=1  dbl_ovrd=off  show_param=off  inserted_by_tool=off  pipeline=off
      settings: xl_area=[0, 0, 0, 0, 0, 0, 0]
  Convert1 : xbsIndex_r3/Convert  arith_type=Boolean  n_bits=8  bin_pt=6  quantization=Truncate  overflow=Wrap  latency=0  explicit_period=off  period=1  dbl_ovrd=off  show_param=off  inserted_by_tool=off  pipeline=off
      settings: xl_area=[0, 0, 0, 0, 0, 0, 0]
  Register1 : xbsIndex_r3/Register  init=0  reg_only_valid=off  explicit_period=on  period=1  rst=off  en=on  out_en=off  dbl_ovrd=off  show_param=off
      settings: xl_area=[0, 0, 0, 0, 0, 0, 0]
  Register23 : xbsIndex_r3/Register  init=0  reg_only_valid=off  explicit_period=on  period=1  rst=off  en=on  out_en=off  dbl_ovrd=off  show_param=off
      settings: xl_area=[0, 0, 0, 0, 0, 0, 0]
  edge1 : xbsIndex_r3/Expression  expression=a & ~b  precision=Full  arith_type=Unsigned  n_bits=8  bin_pt=2  align_bp=on  latency=0  explicit_period=off  period=1  en=off  dbl_ovrd=off  show_param=off
      settings: xl_area=[0, 0, 0, 0, 0, 0, 0]
  q : Outport
  wires:
  Convert1/1 -> edge1/1, Register1/1, Register1/2
  Convert/1 -> Register23/2
  Register1/1 -> edge1/2
  en/1 -> Convert1/1
  edge1/1 -> Convert/1
  d/1 -> Register23/1
  Register23/1 -> q/1

== system t_t_200_tge4/rec/reg_once1 ==
  d : Inport  Port=1  LatchInput=off
  en : Inport  Port=2  LatchInput=off
  Convert : xbsIndex_r3/Convert  arith_type=Boolean  n_bits=8  bin_pt=6  quantization=Truncate  overflow=Wrap  latency=0  explicit_period=off  period=1  dbl_ovrd=off  show_param=off  inserted_by_tool=off  pipeline=off
      settings: xl_area=[0, 0, 0, 0, 0, 0, 0]
  Convert1 : xbsIndex_r3/Convert  arith_type=Boolean  n_bits=8  bin_pt=6  quantization=Truncate  overflow=Wrap  latency=0  explicit_period=off  period=1  dbl_ovrd=off  show_param=off  inserted_by_tool=off  pipeline=off
      settings: xl_area=[0, 0, 0, 0, 0, 0, 0]
  Register1 : xbsIndex_r3/Register  init=0  reg_only_valid=off  explicit_period=on  period=1  rst=off  en=on  out_en=off  dbl_ovrd=off  show_param=off
      settings: xl_area=[0, 0, 0, 0, 0, 0, 0]
  Register23 : xbsIndex_r3/Register  init=0  reg_only_valid=off  explicit_period=on  period=1  rst=off  en=on  out_en=off  dbl_ovrd=off  show_param=off
      settings: xl_area=[0, 0, 0, 0, 0, 0, 0]
  edge1 : xbsIndex_r3/Expression  expression=a & ~b  precision=Full  arith_type=Unsigned  n_bits=8  bin_pt=2  align_bp=on  latency=0  explicit_period=off  period=1  en=off  dbl_ovrd=off  show_param=off
      settings: xl_area=[0, 0, 0, 0, 0, 0, 0]
  q : Outport
  wires:
  Register23/1 -> q/1
  d/1 -> Register23/1
  edge1/1 -> Convert/1
  en/1 -> Convert1/1
  Register1/1 -> edge1/2
  Convert/1 -> Register23/2
  Convert1/1 -> Register1/2, Register1/1, edge1/1

== system t_t_200_tge4/rec/reg_once2 ==
  d : Inport  Port=1  LatchInput=off
  en : Inport  Port=2  LatchInput=off
  Convert : xbsIndex_r3/Convert  arith_type=Boolean  n_bits=8  bin_pt=6  quantization=Truncate  overflow=Wrap  latency=0  explicit_period=off  period=1  dbl_ovrd=off  show_param=off  inserted_by_tool=off  pipeline=off
      settings: xl_area=[0, 0, 0, 0, 0, 0, 0]
  Convert1 : xbsIndex_r3/Convert  arith_type=Boolean  n_bits=8  bin_pt=6  quantization=Truncate  overflow=Wrap  latency=0  explicit_period=off  period=1  dbl_ovrd=off  show_param=off  inserted_by_tool=off  pipeline=off
      settings: xl_area=[0, 0, 0, 0, 0, 0, 0]
  Register1 : xbsIndex_r3/Register  init=0  reg_only_valid=off  explicit_period=on  period=1  rst=off  en=on  out_en=off  dbl_ovrd=off  show_param=off
      settings: xl_area=[0, 0, 0, 0, 0, 0, 0]
  Register23 : xbsIndex_r3/Register  init=0  reg_only_valid=off  explicit_period=on  period=1  rst=off  en=on  out_en=off  dbl_ovrd=off  show_param=off
      settings: xl_area=[0, 0, 0, 0, 0, 0, 0]
  edge1 : xbsIndex_r3/Expression  expression=a & ~b  precision=Full  arith_type=Unsigned  n_bits=8  bin_pt=2  align_bp=on  latency=0  explicit_period=off  period=1  en=off  dbl_ovrd=off  show_param=off
      settings: xl_area=[0, 0, 0, 0, 0, 0, 0]
  q : Outport
  wires:
  Convert1/1 -> edge1/1, Register1/1, Register1/2
  Convert/1 -> Register23/2
  Register1/1 -> edge1/2
  en/1 -> Convert1/1
  edge1/1 -> Convert/1
  d/1 -> Register23/1
  Register23/1 -> q/1

== system t_t_200_tge4/rec/reg_once3 ==
  d : Inport  Port=1  LatchInput=off
  en : Inport  Port=2  LatchInput=off
  Convert : xbsIndex_r3/Convert  arith_type=Boolean  n_bits=8  bin_pt=6  quantization=Truncate  overflow=Wrap  latency=0  explicit_period=off  period=1  dbl_ovrd=off  show_param=off  inserted_by_tool=off  pipeline=off
      settings: xl_area=[0, 0, 0, 0, 0, 0, 0]
  Convert1 : xbsIndex_r3/Convert  arith_type=Boolean  n_bits=8  bin_pt=6  quantization=Truncate  overflow=Wrap  latency=0  explicit_period=off  period=1  dbl_ovrd=off  show_param=off  inserted_by_tool=off  pipeline=off
      settings: xl_area=[0, 0, 0, 0, 0, 0, 0]
  Register1 : xbsIndex_r3/Register  init=0  reg_only_valid=off  explicit_period=on  period=1  rst=off  en=on  out_en=off  dbl_ovrd=off  show_param=off
      settings: xl_area=[0, 0, 0, 0, 0, 0, 0]
  Register23 : xbsIndex_r3/Register  init=0  reg_only_valid=off  explicit_period=on  period=1  rst=off  en=on  out_en=off  dbl_ovrd=off  show_param=off
      settings: xl_area=[0, 0, 0, 0, 0, 0, 0]
  edge1 : xbsIndex_r3/Expression  expression=a & ~b  precision=Full  arith_type=Unsigned  n_bits=8  bin_pt=2  align_bp=on  latency=0  explicit_period=off  period=1  en=off  dbl_ovrd=off  show_param=off
      settings: xl_area=[0, 0, 0, 0, 0, 0, 0]
  q : Outport
  wires:
  Register23/1 -> q/1
  d/1 -> Register23/1
  edge1/1 -> Convert/1
  en/1 -> Convert1/1
  Register1/1 -> edge1/2
  Convert/1 -> Register23/2
  Convert1/1 -> Register1/2, Register1/1, edge1/1

== system t_t_200_tge4/thr/LED_p1event ==
  Sync_In : Inport  Port=1  LatchInput=off
  Scope : Scope
  gpio : xps_library/gpio  Tag=xps:gpio  io_group=BEE2_usr:led  io_dir=out  arith_type=Boolean  bitwidth=1  bin_pt=0  bit_index=2  sample_period=1  use_single_ended=off  use_ddr=off  reg_iob=on  reg_clk_phase=0  termination=None
  wires:
  gpio/1 -> Scope/1
  Sync_In/1 -> gpio/1

== system t_t_200_tge4/thr/LED_p2event ==
  Sync_In : Inport  Port=1  LatchInput=off
  Scope : Scope
  gpio : xps_library/gpio  Tag=xps:gpio  io_group=BEE2_usr:led  io_dir=out  arith_type=Boolean  bitwidth=1  bin_pt=0  bit_index=3  sample_period=1  use_single_ended=off  use_ddr=off  reg_iob=on  reg_clk_phase=0  termination=None
  wires:
  Sync_In/1 -> gpio/1
  gpio/1 -> Scope/1

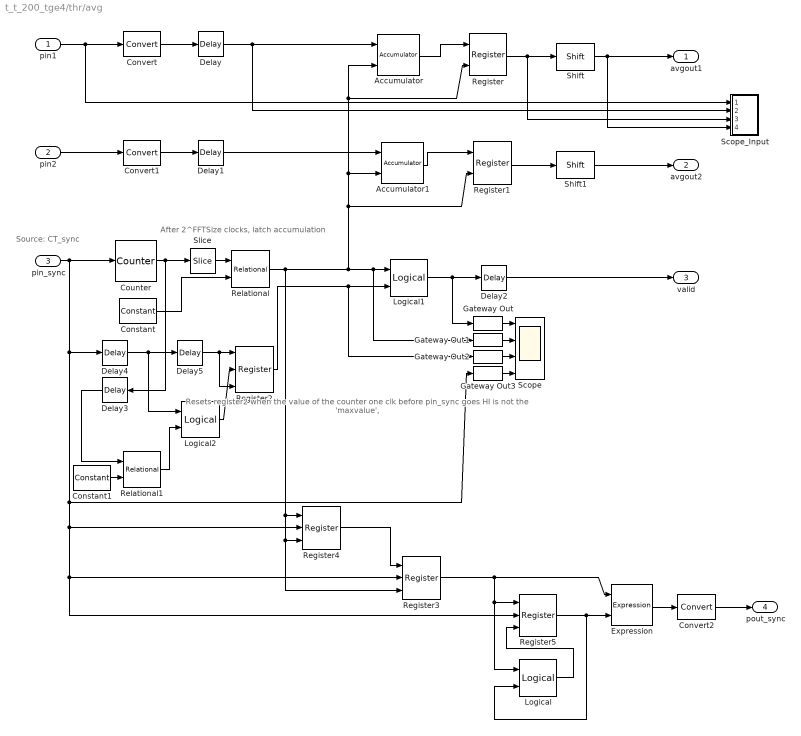
== system t_t_200_tge4/thr/avg ==
  note: After 2^FFTSize clocks,
      | latch accumulation
  note: Resets register2 when
      | the value of the counter
      | one clk before pin_sync goes
      | HI is not the 'maxvalue',
  note: Source: CT_sync
  pin1 : Inport  Port=1  LatchInput=off
  pin2 : Inport  Port=2  LatchInput=off
  pin_sync : Inport  Port=3  LatchInput=off
  Accumulator : xbsIndex_r3/Accumulator  n_bits=FFTSize + 2*DataWidth + 2  overflow=Wrap  operation=Add  scale=1  explicit_period=off  period=1  rst=on  hasbypass=on  en=off  dbl_ovrd=off  show_param=off  gen_core=off  use_rpm=on
      settings: xl_area=[0, 0, 0, 0, 0, 0, 0]
  Accumulator1 : xbsIndex_r3/Accumulator  n_bits=FFTSize + 2*DataWidth + 2  overflow=Wrap  operation=Add  scale=1  explicit_period=off  period=1  rst=on  hasbypass=on  en=off  dbl_ovrd=off  show_param=off  gen_core=off  use_rpm=on
      settings: xl_area=[0, 0, 0, 0, 0, 0, 0]
  Constant : xbsIndex_r3/Constant  const=0  equ=P=C  arith_type=Unsigned  n_bits=FFTSize  bin_pt=0  opselect=C  inp2=PCIN>>17  opr=+  inp1=P  carry=CIN  iostate=0  explicit_period=off  period=1  dbl_ovrd=off
  Constant1 : xbsIndex_r3/Constant  const=2^(FFTSize+PFBSize)-1  equ=P=C  arith_type=Unsigned  n_bits=FFTSize+PFBSize  bin_pt=0  opselect=C  inp2=PCIN>>17  opr=+  inp1=P  carry=CIN  iostate=0  explicit_period=off  period=1  dbl_ovrd=off
  Convert : xbsIndex_r3/Convert  arith_type=Unsigned  n_bits=2*(DataWidth+1) + FFTSize  bin_pt=2*(DataWidth-1)  quantization=Truncate  overflow=Wrap  latency=0  explicit_period=off  period=1  dbl_ovrd=off  show_param=off  inserted_by_tool=off  pipeline=off
      settings: xl_area=[0, 0, 0, 0, 0, 0, 0]
  Convert1 : xbsIndex_r3/Convert  arith_type=Unsigned  n_bits=2*(DataWidth+1) + FFTSize  bin_pt=2*(DataWidth-1)  quantization=Truncate  overflow=Wrap  latency=0  explicit_period=off  period=1  dbl_ovrd=off  show_param=off  inserted_by_tool=off  pipeline=off
      settings: xl_area=[0, 0, 0, 0, 0, 0, 0]
  Convert2 : xbsIndex_r3/Convert  arith_type=Boolean  n_bits=FFTSize + 2*DataWidth + 1  bin_pt=2*DataWidth - 1  quantization=Truncate  overflow=Wrap  latency=0  explicit_period=off  period=1  dbl_ovrd=off  show_param=off  inserted_by_tool=off  pipeline=off
      settings: xl_area=[0, 0, 0, 0, 0, 0, 0]
  Counter : xbsIndex_r3/Counter  cnt_type=Free Running  n_bits=FFTSize+PFBSize  bin_pt=0  arith_type=Unsigned  start_count=0  cnt_to=Inf  cnt_by_val=1  operation=Up  explicit_period=off  period=1  load_pin=off  rst=on  en=off  dbl_ovrd=off  show_param=off  use_rpm=on  gen_core=off
      settings: xl_area=[0, 0, 0, 0, 0, 0, 0]
  Delay{,1..2,4} (4 alike) : xbsIndex_r3/Delay  latency=2  reg_retiming=on  explicit_period=off  period=1  en=off  accept_only_valid=off  init_zero=on  dbl_ovrd=off  show_param=off
      settings: xl_area=[0, 0, 0, 0, 0, 0, 0]
  Delay3 : xbsIndex_r3/Delay  Orientation=left  latency=1  reg_retiming=on  explicit_period=off  period=1  en=off  accept_only_valid=off  init_zero=on  dbl_ovrd=off  show_param=off
      settings: xl_area=[0, 0, 0, 0, 0, 0, 0]
  Delay5 : xbsIndex_r3/Delay  latency=1  reg_retiming=on  explicit_period=off  period=1  en=off  accept_only_valid=off  init_zero=on  dbl_ovrd=off  show_param=off
      settings: xl_area=[0, 0, 0, 0, 0, 0, 0]
  Expression : xbsIndex_r3/Expression  expression=a & ~b  precision=Full  arith_type=Unsigned  n_bits=8  bin_pt=2  align_bp=on  latency=0  explicit_period=off  period=1  en=off  dbl_ovrd=off  show_param=off
      settings: xl_area=[0, 0, 0, 0, 0, 0, 0]
  Gateway Out{,1..3} (4 alike) : xbsIndex_r3/Gateway Out  output_type=Double  nbits=8  bin_pt=6  arith_type=Boolean  quantization=Truncate  overflow=Wrap  hdl_port=off  timing_constraint=None  locs_specified=off  LOCs={}  needs_fixed_name=off  show_param=off
      settings: xl_area=[0, 0, 0, 0, 0, 0, 0]
  Logical : xbsIndex_r3/Logical  logical_function=XOR  inputs=2  precision=Full  arith_type=Unsigned  n_bits=8  bin_pt=2  align_bp=on  latency=0  explicit_period=off  period=1  en=off  dbl_ovrd=off  show_param=off
      settings: xl_area=[0, 0, 0, 0, 0, 0, 0]
  Logical1 : xbsIndex_r3/Logical  logical_function=AND  inputs=2  precision=Full  arith_type=Unsigned  n_bits=8  bin_pt=2  align_bp=on  latency=0  explicit_period=off  period=1  en=off  dbl_ovrd=off  show_param=off
      settings: xl_area=[0, 0, 0, 0, 0, 0, 0]
  Logical2 : xbsIndex_r3/Logical  logical_function=AND  inputs=2  precision=Full  arith_type=Unsigned  n_bits=8  bin_pt=2  align_bp=on  latency=0  explicit_period=off  period=1  en=off  dbl_ovrd=off  show_param=off
      settings: xl_area=[0, 0, 0, 0, 0, 0, 0]
  Register : xbsIndex_r3/Register  init=0  reg_only_valid=off  explicit_period=off  period=1  rst=off  en=on  out_en=off  dbl_ovrd=off  show_param=off
      settings: xl_area=[0, 0, 0, 0, 0, 0, 0]
  Register1 : xbsIndex_r3/Register  init=0  reg_only_valid=off  explicit_period=off  period=1  rst=off  en=on  out_en=off  dbl_ovrd=off  show_param=off
      settings: xl_area=[0, 0, 0, 0, 0, 0, 0]
  Register2 : xbsIndex_r3/Register  init=0  reg_only_valid=off  explicit_period=off  period=1  rst=on  en=on  out_en=off  dbl_ovrd=off  show_param=off
      settings: xl_area=[0, 0, 0, 0, 0, 0, 0]
  Register3 : xbsIndex_r3/Register  init=0  reg_only_valid=off  explicit_period=off  period=1  rst=on  en=on  out_en=off  dbl_ovrd=off  show_param=off
      settings: xl_area=[0, 0, 0, 0, 0, 0, 0]
  Register4 : xbsIndex_r3/Register  init=0  reg_only_valid=off  explicit_period=off  period=1  rst=on  en=on  out_en=off  dbl_ovrd=off  show_param=off
      settings: xl_area=[0, 0, 0, 0, 0, 0, 0]
  Register5 : xbsIndex_r3/Register  init=0  reg_only_valid=off  explicit_period=on  period=1  rst=on  en=on  out_en=off  dbl_ovrd=off  show_param=off
      settings: xl_area=[0, 0, 0, 0, 0, 0, 0]
  Relational : xbsIndex_r3/Relational  mode=a=b  latency=2  explicit_period=off  period=1  en=off  dbl_ovrd=off  show_param=off
      settings: xl_area=[0, 0, 0, 0, 0, 0, 0]
  Relational1 : xbsIndex_r3/Relational  mode=a!=b  latency=1  explicit_period=off  period=1  en=off  dbl_ovrd=off  show_param=off
      settings: xl_area=[0, 0, 0, 0, 0, 0, 0]
  Scope : Scope  NumInputPorts=4
      settings: YMin=-5~-5~-5~-5  YMax=5~5~5~5  SaveName=ScopeData11
  Scope_Input : Subsystem
  Shift : xbsIndex_r3/Shift  shift_dir=Right  shift_bits=FFTSize  precision=User Defined  arith_type=Unsigned  n_bits=2*DataWidth + 1  bin_pt=2*(DataWidth - 1)  quantization=Truncate  overflow=Wrap  latency=1  explicit_period=off  period=1  en=off  dbl_ovrd=off  show_param=off
      settings: xl_area=[0, 0, 0, 0, 0, 0, 0]
  Shift1 : xbsIndex_r3/Shift  shift_dir=Right  shift_bits=FFTSize  precision=User Defined  arith_type=Unsigned  n_bits=2*DataWidth + 1  bin_pt=2*(DataWidth - 1)  quantization=Truncate  overflow=Wrap  latency=1  explicit_period=off  period=1  en=off  dbl_ovrd=off  show_param=off
      settings: xl_area=[0, 0, 0, 0, 0, 0, 0]
  Slice : xbsIndex_r3/Slice  mode=Lower Bit Location + Width  nbits=FFTSize  bit1=0  base1=MSB of Input  bit0=0  base0=LSB of Input  boolean_output=off  explicit_period=off  period=1  dbl_ovrd=off
  avgout1 : Outport
  avgout2 : Outport  Port=2
  valid : Outport  Port=3
  pout_sync : Outport  Port=4
  wires:
  Gateway Out2/1 -> Scope/3
  Gateway Out1/1 -> Scope/2
  Gateway Out/1 -> Scope/1
  Delay5/1 -> Register2/3, Register2/1
  Delay3/1 -> Relational1/1
  Constant1/1 -> Relational1/2
  Relational1/1 -> Logical2/2
  Logical2/1 -> Register2/2
  Slice/1 -> Relational/1
  Delay4/1 -> Delay5/1, Logical2/1
  Register2/1 -> Gateway Out2/1, Logical1/2
  Convert2/1 -> pout_sync/1
  Register4/1 -> Register3/1
  Expression/1 -> Convert2/1
  Register3/1 -> Register5/1, Logical/1, Expression/1
  Logical/1 -> Register5/3
  Register5/1 -> Logical/2, Expression/2
  Logical1/1 -> Gateway Out/1, Delay2/1
  Relational/1 -> Register3/3, Register4/3, Register4/1, Gateway Out1/1, Logical1/1, Accumulator/2, Register/2, Accumulator1/2, Register1/2
  pin1/1 -> Scope_Input/1(DataA), Convert/1
  pin2/1 -> Convert1/1
  Convert/1 -> Delay/1
  pin_sync/1 -> Delay4/1, Register5/2, Register3/2, Register4/2, Gateway Out3/1, Counter/1
  Counter/1 -> Delay3/1, Slice/1
  Constant/1 -> Relational/2
  Delay/1 -> Scope_Input/2(DataB), Accumulator/1
  Accumulator/1 -> Register/1
  Register/1 -> Scope_Input/3(DataC), Shift/1
  Shift/1 -> Scope_Input/4(Sync), avgout1/1
  Convert1/1 -> Delay1/1
  Delay1/1 -> Accumulator1/1
  Accumulator1/1 -> Register1/1
  Register1/1 -> Shift1/1
  Shift1/1 -> avgout2/1
  Delay2/1 -> valid/1
  Gateway Out3/1 -> Scope/4
